simulink model "sfcndemo_sfun_zc"  (Simulink 6.0)
settings: Solver=FixedStepDiscrete  StartTime=0.0  StopTime=10.0  RelTol=1e-3
settings Model: Creator=The MathWorks Inc.  LastModifiedBy=batserve  ExtModeTrigMode=oneshot  ExtModeArmWhenConnect=off  ExtModeAutoUpdateStatusClock=off
settings DataIOCC: LimitDataPoints=off
settings OptimizationCC: BooleanDataType=off
settings DebuggingCC: CheckExecutionContextPreStartOutputMsg=on  CheckExecutionContextRuntimeOutputMsg=on  SolverPrmCheckMsg=none
settings HardwareCC: TargetUnknown=on
settings RTWCC: TemplateMakefile=grt_vc.tmf

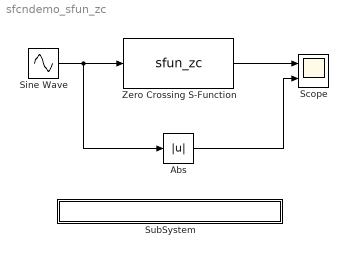
== system sfcndemo_sfun_zc ==
  Abs : Abs  SaturateOnIntegerOverflow=on
  Scope : Scope  NumInputPorts=2
      settings: TimeRange=10  YMin=0~0  YMax=2~2
  Sine Wave : Sin  Amplitude=1:2  SampleTime=0
  SubSystem : Subsystem  PropExecContextAcrossSSBoundary=on
      settings: OpenFcn=edit(fullfile(matlabroot,'simulink','src','sfun_zc.c'))
      mask Display: disp('matlabroot\simulink\src\sfun_zc.c');
  Zero Crossing S-Function : S-Function  FunctionName=sfun_zc
      mask Type: S-function: sfun_zc
      mask Description: This is a S-function block which has nonsampled zero crossings.
  wires:
  Zero Crossing S-Function/1 -> Scope/1
  Abs/1 -> Scope/2
  Sine Wave/1 -> Zero Crossing S-Function/1, Abs/1

== system sfcndemo_sfun_zc/SubSystem ==
